simulink subsystem "Main_Kalman_2D"  (R2024a)
settings: Solver=VariableStepAuto  StartTime=0.0  StopTime=10.0  RelTol=1e-3
settings Model: Creator=Peter  LastModifiedBy=Peter

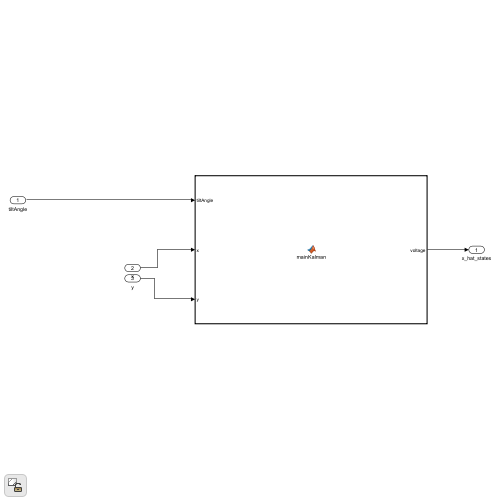
[thumbnail: Simulink's stored preview of the top-level diagram]
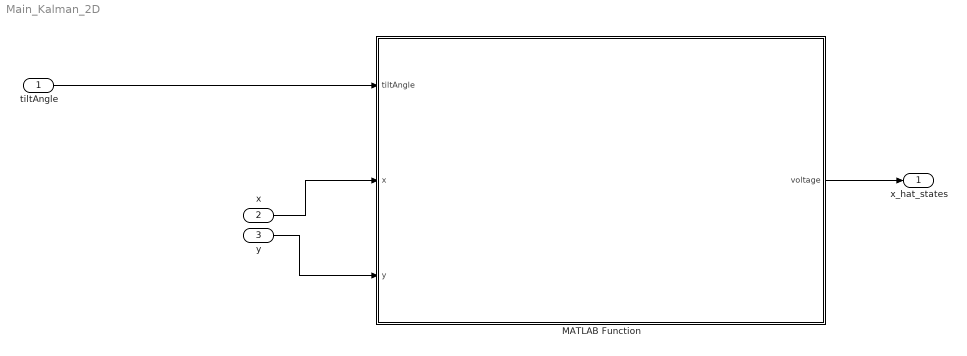
== system Main_Kalman_2D ==
  tiltAngle : Inport
  x : Inport  Port=2
  y : Inport  Port=3
  MATLAB Function : MATLAB Function  TreatAsAtomicUnit=on
  x_hat_states : Outport
  wires:
  y/1 -> MATLAB Function/3(y)
  tiltAngle/1 -> MATLAB Function/1(tiltAngle)
  x/1 -> MATLAB Function/2(x)
  MATLAB Function/1(voltage) -> x_hat_states/1

== matlab function Main_Kalman_2D/MATLAB Function ==
  data: tiltAngle input single; voltage output; x input single; y input single
function voltage = mainKalman(tiltAngle, x, y)

voltage = 1;
